simulink model "obsvSimul"  (R2014a)
settings: Solver=ode45  StartTime=0.0  StopTime=25  RelTol=1e-3
undefined symbols (not defined in the file or in its folder): A, B, C, F, G, Kd, L, x0, x_esht_0
settings Model: Creator=dimpa  LastModifiedBy=dimpa

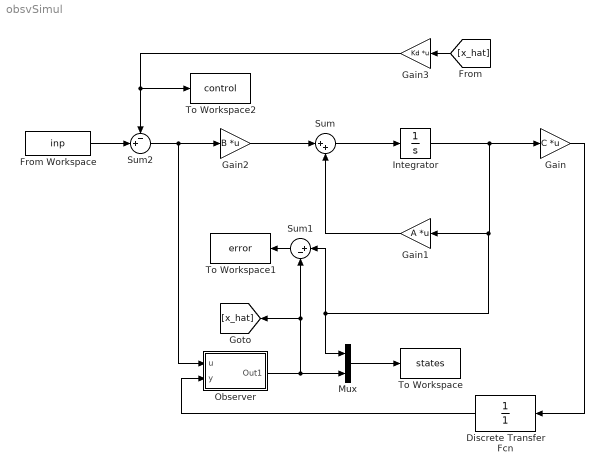
== system obsvSimul ==
  Discrete Transfer Fcn : DiscreteTransferFcn  Denominator=[1]  SampleTime=0.1
  From Workspace : FromWorkspace  VariableName=inp  SampleTime=0.1
  Gain : Gain  Gain=C  Multiplication=Matrix(K*u) (u vector)
  Gain1 : Gain  Gain=A  Multiplication=Matrix(K*u) (u vector)
  Gain2 : Gain  Gain=B  Multiplication=Matrix(K*u) (u vector)
  Gain3 : Gain  Gain=Kd  Multiplication=Matrix(K*u) (u vector)
  Integrator : Integrator  InitialCondition=x0
  Mux : Mux  Inputs=2
  Observer : Subsystem
  Sum : Sum  Inputs=|++
  Sum1 : Sum  Inputs=|+-
  Sum2 : Sum  Inputs=-+|
  To Workspace : ToWorkspace  VariableName=states  SaveFormat=Structure With Time  SampleTime=-1
  To Workspace1 : ToWorkspace  VariableName=error  SaveFormat=Structure With Time  SampleTime=-1
  To Workspace2 : ToWorkspace  VariableName=control  SaveFormat=Structure With Time  SampleTime=-1
  wires:
  Gain2/1 -> Sum/1
  Sum/1 -> Integrator/1
  Gain1/1 -> Sum/2
  Gain/1 -> Discrete Transfer Fcn/1
  Sum2/1 -> Observer/1(u), Gain2/1
  Observer/1(Out1) -> Mux/2, [x_hat], Sum1/2
  Mux/1 -> To Workspace/1
  Integrator/1 -> Sum1/1, Mux/1, Gain1/1, Gain/1
  Discrete Transfer Fcn/1 -> Observer/2(y)
  Sum1/1 -> To Workspace1/1
  [x_hat] -> Gain3/1
  From Workspace/1 -> Sum2/2
  Gain3/1 -> To Workspace2/1, Sum2/1

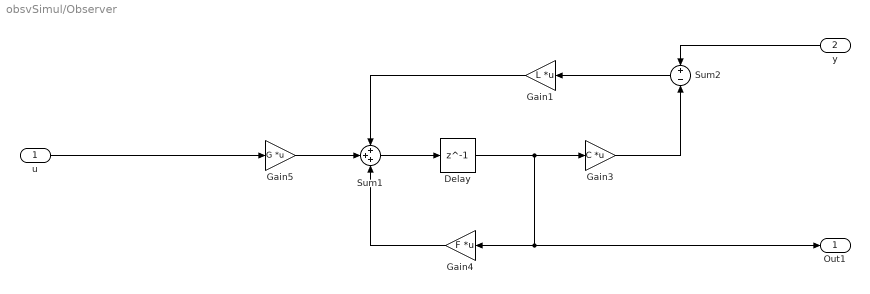
== system obsvSimul/Observer ==
  u : Inport
  y : Inport  Port=2
  Delay : Delay  DelayLength=1  InitialCondition=x_esht_0  SampleTime=0.1
  Gain1 : Gain  Gain=L  Multiplication=Matrix(K*u) (u vector)
  Gain3 : Gain  Gain=C  Multiplication=Matrix(K*u) (u vector)
  Gain4 : Gain  Gain=F  Multiplication=Matrix(K*u) (u vector)
  Gain5 : Gain  Gain=G  Multiplication=Matrix(K*u) (u vector)
  Sum1 : Sum  Inputs=+++
  Sum2 : Sum  Inputs=+-
  Out1 : Outport
  wires:
  Gain5/1 -> Sum1/2
  Sum1/1 -> Delay/1
  Delay/1 -> Gain3/1, Out1/1, Gain4/1
  Gain4/1 -> Sum1/3
  Gain3/1 -> Sum2/2
  u/1 -> Gain5/1
  y/1 -> Sum2/1
  Sum2/1 -> Gain1/1
  Gain1/1 -> Sum1/1
